simulink model "ParallelProcessing"  (Simulink 7.7)
settings: Solver=ode45  StartTime=0.0  StopTime=inf  RelTol=1e-3
settings Model: Creator=Birdman  LastModifiedBy=Birdman

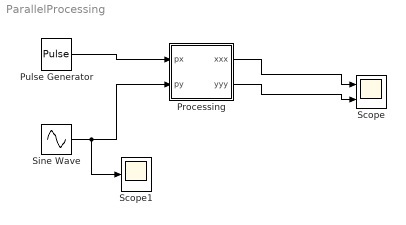
== system ParallelProcessing ==
  Processing : Stateflow chart  TreatAsAtomicUnit=on
  Pulse Generator : DiscretePulseGenerator  PulseType=Time based  Period=1  PulseWidth=50
  Scope : Scope  NumInputPorts=2
      settings: YMin=5~-11  YMax=6~-9
  Scope1 : Scope
      settings: YMin=-1  YMax=1
  Sine Wave : Sin  SampleTime=0
  wires:
  Processing/1(xxx) -> Scope/1
  Processing/2(yyy) -> Scope/2
  Pulse Generator/1 -> Processing/1(px)
  Sine Wave/1 -> Processing/2(py), Scope1/1

== stateflow chart Processing ==
  settings: sampleTime=0.05
  state DAQ [parallel]
    settings: executionOrder=1
    state daq
      en: i=0;
      du: x[i]=px; y[i]=py; i++;
      ex: xx=x; yy=y;
    (default) -> daq
    daq -> daq : [i==20]/send(DataReady,Calculation)
  state Calculation [parallel]
    settings: executionOrder=2
    state shift
      en: xxx=avg(xx); yyy=avg(yy);
    state Standby
    shift -> Standby
    (default) -> Standby
    Standby -> shift : DataReady
  data: u function_input double size=20; v function_output double size=1; px input double; py input double; x local double size=20 =0; y local double size=20 =0; xx local double size=20 =0; yy local double size=20 =0; xxx output double size=1 =0; yyy output double size=1 =0; i local double
  events: DataReady local EITHER_EDGE_EVENT
  function v=avg(u):
    | function v=avg(u)
    |  
    | v=mean(u);
